simulink model "simulink_controlehinf"  (R2018a)
settings: Solver=ode45  StartTime=0.0  StopTime=100  RelTol=1e-3  EnableMultiTasking=on
values from neighbouring files (symbols this model uses):
  Ts = 0.5    [Ball_In_Tube.m]
undefined symbols (not defined in the file or in its folder): K2
settings Model: Creator=uidv5645  LastModifiedBy=uidv5645
settings DataIOCC: LimitDataPoints=on  SaveFormat=Array
settings OptimizationCC: LifeSpan=inf
settings DebuggingCC: SFUnexpectedBacktrackingDiag=warning  SFNoUnconditionalDefaultTransitionDiag=warning  SFExecutionAtInitializationDiag=none
settings HardwareCC: ProdBitPerPointer=32  ProdBitPerSizeT=32  ProdBitPerPtrDiffT=32  ProdLargestAtomicFloat=None  ProdIntDivRoundTo=Undefined  ProdEndianess=Unspecified  ProdWordSize=32  ProdHWDeviceType=32-bit Generic
settings ModelReferenceCC: PropagateSignalLabelsOutOfModel=off
settings CodeAppCC: StateflowObjectComments=on
settings GRTTargetCC: TargetLangStandard=C89/C90 (ANSI)  GeneratePreprocessorConditionals=Disable all
settings ConfigComp: CovMetricSettings=dw  CovHtmlReporting=on  CovSaveCumulativeToWorkspaceVar=on  CovSaveSingleToWorkspaceVar=on  CovExternalEMLEnable=off

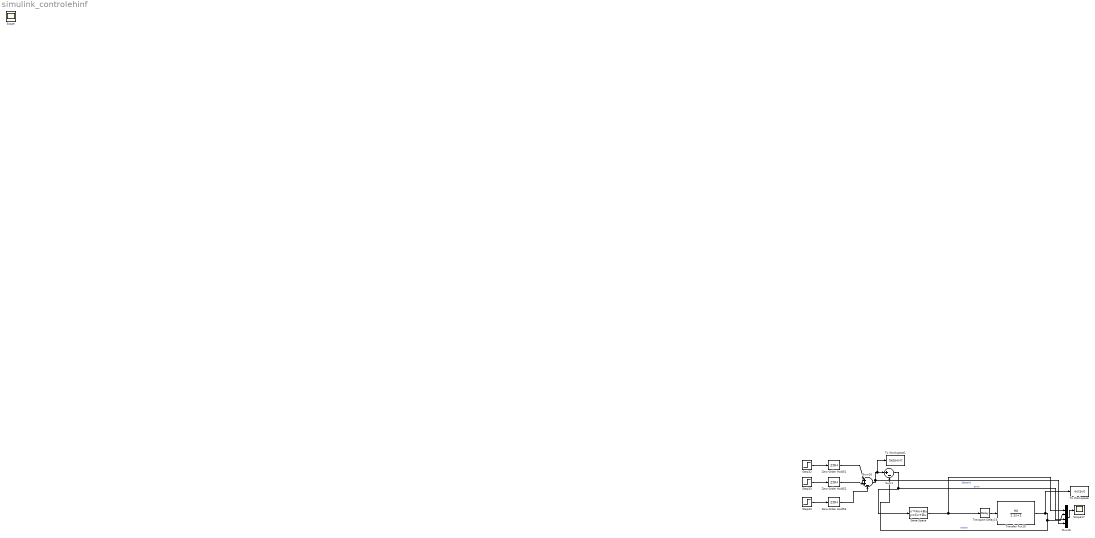
== system simulink_controlehinf ==
  Mux16 : Mux
  Scope17 : Scope
  State-Space : StateSpace  A=K2.A  B=K2.B  C=K2.C  D=K2.D  InitialCondition=0
  Step32 : Step  Time=70  After=20  SampleTime=0.05
  Step33 : Step  After=70  SampleTime=0.05
  Step34 : Step  Time=40  After=40  SampleTime=Ts
  Sum1 : Sum  Inputs=|+-
  Sum16 : Sum  Inputs=|++-
  To Workspace : ToWorkspace  VariableName=output  SaveFormat=Timeseries  SampleTime=-1
  To Workspace1 : ToWorkspace  VariableName=Setpoint  SaveFormat=Timeseries  SampleTime=-1
  Transfer Fcn19 : TransferFcn  Numerator=[90]  Denominator=[1.1 1]
  Transport Delay16 : TransportDelay  DelayTime=1.25
  Zero-Order Hold51 : ZeroOrderHold  SampleTime=Ts
  Zero-Order Hold52 : ZeroOrderHold  SampleTime=Ts
  Zero-Order Hold53 : ZeroOrderHold  SampleTime=Ts
  Scope : Scope
  wires:
  Mux16/1 -> Scope17/1
  Zero-Order Hold51/1 -> Sum16/1
  Transfer Fcn19/1 -> To Workspace/1, Sum1/2, Mux16/2  "output"
  Transport Delay16/1 -> Transfer Fcn19/1
  Step32/1 -> Zero-Order Hold51/1
  State-Space/1 -> Transport Delay16/1, Mux16/1
  Sum16/1 -> Mux16/4, To Workspace1/1, Sum1/1  "Setpoint"
  Step33/1 -> Zero-Order Hold52/1
  Step34/1 -> Zero-Order Hold53/1
  Zero-Order Hold53/1 -> Sum16/3
  Zero-Order Hold52/1 -> Sum16/2
  Sum1/1 -> State-Space/1, Mux16/3  "error"
